simulink model "RMIC_ident_experiment"  (R2020a)
settings: Solver=ode4  StartTime=0.0  StopTime=30  FixedStep=1e-3  RelTol=1e-3
values from neighbouring files (symbols this model uses):
  lambdas = RMIC_get_fourier_lambdas(constPar.a_test, constPar.noj, constPar.nop, constPar.tend, constPar.omega, constPar.q_bound, constPar)    [RMIC_ident_experiment_start.m]
  q_dist_var = (pi*0.005/2)^2    (= 6.16850275068e-05)    [RMIC_ident_experiment_start.m]
  seed = 0    [RMIC_ident_experiment_start.m]
  T_smp = 1E-3    (= 0.001)    [RMIC_ident_experiment_start.m]
undefined symbols (not defined in the file or in its folder): constPar, f_c, f_nu, g, I1zz, I2zz, l1, lc1, lc2, m1, m2
settings Model: Creator=Tenghu  LastModifiedBy=fernando
settings SolverCC: ZeroCrossControl=EnableAll  AlgebraicLoopSolver=LineSearch
settings DataIOCC: SaveFormat=StructureWithTime
settings OptimizationCC: BlockReduction=off  BooleanDataType=off  LifeSpan=inf
settings DebuggingCC: SaveWithParameterizedLinksMsg=none  UnderspecifiedInitializationDetection=Classic  MergeDetectMultiDrivingBlocksExec=none  SignalResolutionControl=TryResolveAllWithWarning  AllowSymbolicDim=off  SFUnexpectedBacktrackingDiag=warning  SFNoUnconditionalDefaultTransitionDiag=warning  SFExecutionAtInitializationDiag=none  ArithmeticOperatorsInVariantConditions=warning
settings HardwareCC: ProdBitPerPointer=32  ProdBitPerSizeT=32  ProdBitPerPtrDiffT=32  ProdLargestAtomicFloat=None  ProdIntDivRoundTo=Undefined  ProdEndianess=Unspecified  ProdWordSize=32  ProdHWDeviceType=32-bit Generic  TargetBitPerLong=64  TargetBitPerPointer=64  TargetBitPerSizeT=64  TargetBitPerPtrDiffT=64  TargetLongLongMode=on  TargetIntDivRoundTo=Zero  TargetEndianess=LittleEndian  TargetWordSize=64  TargetHWDeviceType=MATLAB Host  ProdEqTarget=off
settings ModelReferenceCC: PropagateSignalLabelsOutOfModel=off
settings SFSimCC: SimUseLocalCustomCode=off  CustomCodeUndefinedFunction=UseInterfaceOnly
settings RTWCC: RTWUseLocalCustomCode=off
settings CodeAppCC: StateflowObjectComments=on
settings GRTTargetCC: TargetLangStandard=C89/C90 (ANSI)
settings ConfigComp: CovMetricSettings=dw  CovHtmlReporting=on  CovSaveCumulativeToWorkspaceVar=on  CovSaveSingleToWorkspaceVar=on  CovExternalEMLEnable=off  CovSFcnEnable=off

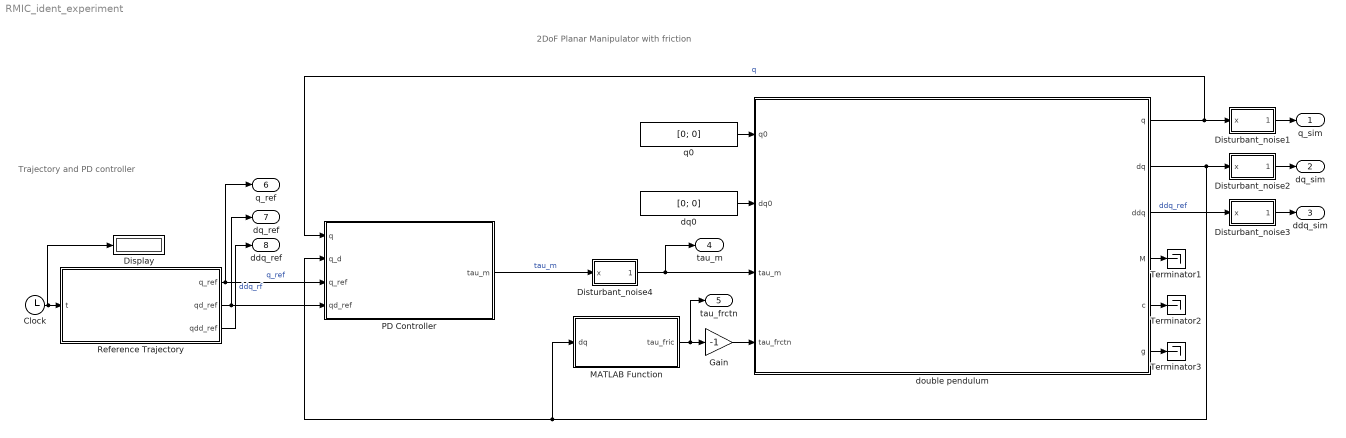
== system RMIC_ident_experiment ==
  note: Trajectory and PD controller
  note: 2DoF Planar Manipulator with friction
  Clock : Clock
  Display : Display
  Disturbant_noise1 : Subsystem  mask{q_dist_var=q_dist_var*100}
      mask prompts: q_dist_var "Varaiance of noise [rad^2]"
  Disturbant_noise2 : Subsystem  mask{q_dist_var=q_dist_var*100*2*pi}
      mask prompts: q_dist_var "Varaiance of noise [rad^2]"
  Disturbant_noise3 : Subsystem  mask{q_dist_var=q_dist_var*100*6*pi^2}
      mask prompts: q_dist_var "Varaiance of noise [rad^2]"
  Disturbant_noise4 : Subsystem  mask{q_dist_var=1.5^2}
      mask prompts: q_dist_var "Varaiance of noise [rad^2]"
  Gain : Gain  Gain=-1
  MATLAB Function : MATLAB Function  TreatAsAtomicUnit=on
  PD Controller : Subsystem
      mask Display:
      | image(imread('./controller.png'))
      | port_label('input', 1, 'q','interpreter','tex')
      | port_label('input', 2, 'dq','interpreter','tex')
      | port_label('input', 3, 'q_{ref}','interpreter','tex')
      | port_label('input', 4, 'dq_{ref}','interpreter','tex')
      | port_label('output', 1, '\tau_m','interpreter','tex')
  Reference Trajectory : Subsystem
      mask Display:
      | image(imread('./trajectory.png'))
      | port_label('input', 1, 't','interpreter','tex')
      | port_label('output', 1, 'q_{ref}','interpreter','tex')
      | port_label('output', 2, 'dq{ref}','interpreter','tex')
      | port_label('output', 3, 'ddq{ref}','interpreter','tex')
  Terminator1 : Terminator
  Terminator2 : Terminator
  Terminator3 : Terminator
  double pendulum : Subsystem
      mask Display:
      | image(imread('./double_pendulum.png'))
      | port_label('input', 1, 'q_0','interpreter','tex')
      | port_label('input', 2, 'dq_0','interpreter','tex')
      | port_label('input', 3, 'tau_{m}','interpreter','tex')
      | port_label('input', 4, 'tau_{frctn}','interpreter','tex')
      | 
      | port_label('output', 1, 'q','interpreter','tex')
      | port_label('output', 2, 'dq','interpreter','tex')
      | port_label('output', 3, 'ddq','interpreter','tex')
      | port_label('output', 4, 'M(q)','interpreter','tex')
      | port_label('output', 5, 'c(q,dq)','interpreter','tex')
      | port_label('output', 6, 'g(q)')
  dq0 : Constant  Value=[0; 0]
  q0 : Constant  Value=[0; 0]
  q_sim : Outport  VectorParamsAs1DForOutWhenUnconnected=off
  dq_sim : Outport  Port=2  VectorParamsAs1DForOutWhenUnconnected=off
  ddq_sim : Outport  Port=3  VectorParamsAs1DForOutWhenUnconnected=off
  tau_m : Outport  Port=4  VectorParamsAs1DForOutWhenUnconnected=off
  tau_frctn : Outport  Port=5  VectorParamsAs1DForOutWhenUnconnected=off
  q_ref : Outport  Port=6  VectorParamsAs1DForOutWhenUnconnected=off
  dq_ref : Outport  Port=7  VectorParamsAs1DForOutWhenUnconnected=off
  ddq_ref : Outport  Port=8  VectorParamsAs1DForOutWhenUnconnected=off
  wires:
  double pendulum/4(M) -> Terminator1/1
  double pendulum/5(c) -> Terminator2/1
  double pendulum/6(g) -> Terminator3/1
  dq0/1 -> double pendulum/2(dq0)
  q0/1 -> double pendulum/1(q0)
  Clock/1 -> Display/1, Reference Trajectory/1(t)
  MATLAB Function/1(tau_fric) -> tau_frctn/1, Gain/1
  double pendulum/3(ddq) -> Disturbant_noise3/1(x)  "ddq_ref"
  double pendulum/2(dq) -> Disturbant_noise2/1(x), MATLAB Function/1(dq), PD Controller/2(q_d)
  Gain/1 -> double pendulum/4(tau_frctn)
  PD Controller/1(tau_m) -> Disturbant_noise4/1(x)  "tau_m"
  double pendulum/1(q) -> Disturbant_noise1/1(x), PD Controller/1(q)  "q"
  Disturbant_noise2/1(x_dist) -> dq_sim/1
  Disturbant_noise1/1(x_dist) -> q_sim/1
  Disturbant_noise3/1(x_dist) -> ddq_sim/1
  Disturbant_noise4/1(x_dist) -> tau_m/1, double pendulum/3(tau_m)
  Reference Trajectory/3(qdd_ref) -> ddq_ref/1  "ddq_rf"
  Reference Trajectory/1(q_ref) -> q_ref/1, PD Controller/3(q_ref)  "q_ref"
  Reference Trajectory/2(qd_ref) -> dq_ref/1, PD Controller/4(qd_ref)

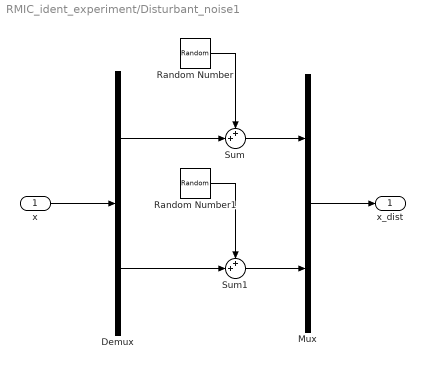
== system RMIC_ident_experiment/Disturbant_noise1 ==
  x : Inport
  Demux : Demux  Outputs=2
  Mux : Mux  Inputs=2
  Random Number : RandomNumber  Variance=q_dist_var  Seed=seed  SampleTime=T_smp
  Random Number1 : RandomNumber  Variance=q_dist_var  Seed=seed  SampleTime=T_smp
  Sum : Sum  Inputs=++|
  Sum1 : Sum  Inputs=++|
  x_dist : Outport  VectorParamsAs1DForOutWhenUnconnected=off
  wires:
  Sum/1 -> Mux/1
  Sum1/1 -> Mux/2
  Mux/1 -> x_dist/1
  x/1 -> Demux/1
  Random Number1/1 -> Sum1/1
  Random Number/1 -> Sum/1
  Demux/1 -> Sum/2
  Demux/2 -> Sum1/2

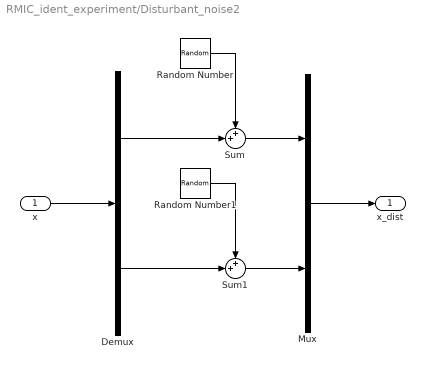
== system RMIC_ident_experiment/Disturbant_noise2 ==
  x : Inport
  Demux : Demux  Outputs=2
  Mux : Mux  Inputs=2
  Random Number : RandomNumber  Variance=q_dist_var  Seed=seed  SampleTime=T_smp
  Random Number1 : RandomNumber  Variance=q_dist_var  Seed=seed  SampleTime=T_smp
  Sum : Sum  Inputs=++|
  Sum1 : Sum  Inputs=++|
  x_dist : Outport  VectorParamsAs1DForOutWhenUnconnected=off
  wires:
  Sum/1 -> Mux/1
  Sum1/1 -> Mux/2
  Mux/1 -> x_dist/1
  x/1 -> Demux/1
  Random Number1/1 -> Sum1/1
  Random Number/1 -> Sum/1
  Demux/1 -> Sum/2
  Demux/2 -> Sum1/2

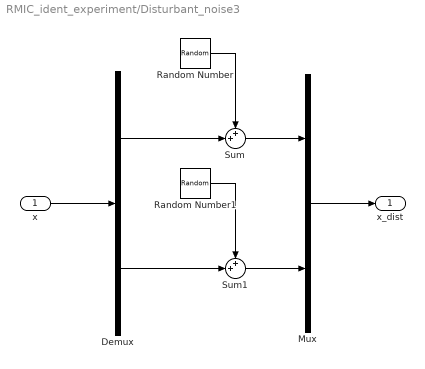
== system RMIC_ident_experiment/Disturbant_noise3 ==
  x : Inport
  Demux : Demux  Outputs=2
  Mux : Mux  Inputs=2
  Random Number : RandomNumber  Variance=q_dist_var  Seed=seed  SampleTime=T_smp
  Random Number1 : RandomNumber  Variance=q_dist_var  Seed=seed  SampleTime=T_smp
  Sum : Sum  Inputs=++|
  Sum1 : Sum  Inputs=++|
  x_dist : Outport  VectorParamsAs1DForOutWhenUnconnected=off
  wires:
  Sum/1 -> Mux/1
  Sum1/1 -> Mux/2
  Mux/1 -> x_dist/1
  x/1 -> Demux/1
  Random Number1/1 -> Sum1/1
  Random Number/1 -> Sum/1
  Demux/1 -> Sum/2
  Demux/2 -> Sum1/2

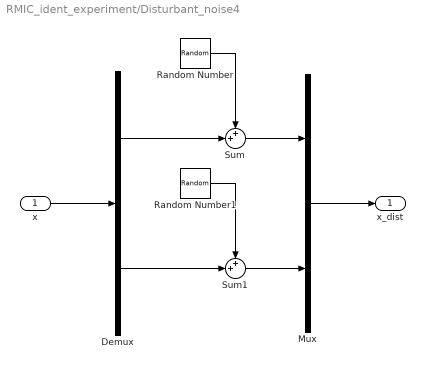
== system RMIC_ident_experiment/Disturbant_noise4 ==
  x : Inport
  Demux : Demux  Outputs=2
  Mux : Mux  Inputs=2
  Random Number : RandomNumber  Variance=q_dist_var  Seed=seed  SampleTime=T_smp
  Random Number1 : RandomNumber  Variance=q_dist_var  Seed=seed  SampleTime=T_smp
  Sum : Sum  Inputs=++|
  Sum1 : Sum  Inputs=++|
  x_dist : Outport  VectorParamsAs1DForOutWhenUnconnected=off
  wires:
  Demux/1 -> Sum/2
  Sum/1 -> Mux/1
  Demux/2 -> Sum1/2
  Sum1/1 -> Mux/2
  Random Number1/1 -> Sum1/1
  x/1 -> Demux/1
  Mux/1 -> x_dist/1
  Random Number/1 -> Sum/1

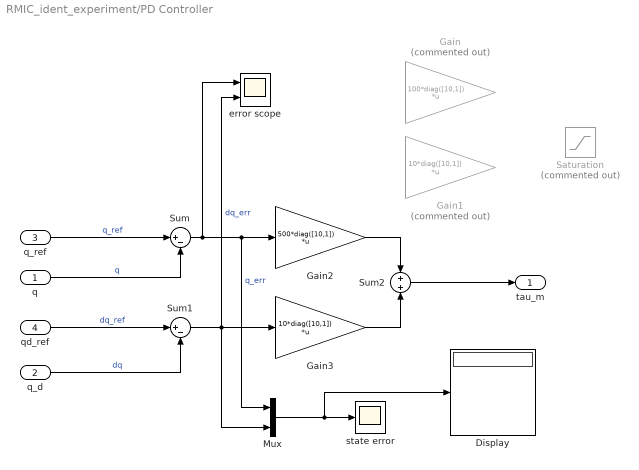
== system RMIC_ident_experiment/PD Controller ==
  q : Inport
  q_d : Inport  Port=2
  q_ref : Inport  Port=3
  qd_ref : Inport  Port=4
  Display : Display
  Gain : Gain  Commented=on  Gain=100*diag([10,1])  Multiplication=Matrix(K*u)
  Gain1 : Gain  Commented=on  Gain=10*diag([10,1])  Multiplication=Matrix(K*u)
  Gain2 : Gain  Gain=500*diag([10,1])  Multiplication=Matrix(K*u)
  Gain3 : Gain  Gain=10*diag([10,1])  Multiplication=Matrix(K*u)
  Mux : Mux  Inputs=2
  Saturation : Saturate  Commented=on  UpperLimit=constPar.maxTorque  LowerLimit=constPar.minTorque
  Sum : Sum  Inputs=|+-
  Sum1 : Sum  Inputs=|+-
  Sum2 : Sum
  error scope : Scope  NumInputPorts=2
  state error : Scope
  tau_m : Outport  VectorParamsAs1DForOutWhenUnconnected=off
  wires:
  q_ref/1 -> Sum/1  "q_ref"
  Sum/1 -> error scope/1, Gain2/1, Mux/1  "q_err"
  Sum1/1 -> Gain3/1, Mux/2, error scope/2  "dq_err"
  q/1 -> Sum/2  "q"
  q_d/1 -> Sum1/2  "dq"
  Mux/1 -> Display/1, state error/1
  Gain2/1 -> Sum2/1
  Gain3/1 -> Sum2/2
  Sum2/1 -> tau_m/1
  qd_ref/1 -> Sum1/1  "dq_ref"

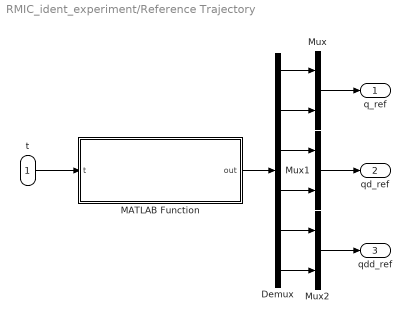
== system RMIC_ident_experiment/Reference Trajectory ==
  t : Inport
  Demux : Demux  Outputs=6
  MATLAB Function : MATLAB Function  TreatAsAtomicUnit=on
  Mux : Mux  Inputs=2
  Mux1 : Mux  Inputs=2
  Mux2 : Mux  Inputs=2
  q_ref : Outport  VectorParamsAs1DForOutWhenUnconnected=off
  qd_ref : Outport  Port=2  VectorParamsAs1DForOutWhenUnconnected=off
  qdd_ref : Outport  Port=3  VectorParamsAs1DForOutWhenUnconnected=off
  wires:
  t/1 -> MATLAB Function/1(t)
  Demux/1 -> Mux/1
  Demux/2 -> Mux/2
  Demux/3 -> Mux1/1
  Demux/4 -> Mux1/2
  Demux/5 -> Mux2/1
  Demux/6 -> Mux2/2
  MATLAB Function/1(out) -> Demux/1
  Mux/1 -> q_ref/1
  Mux1/1 -> qd_ref/1
  Mux2/1 -> qdd_ref/1

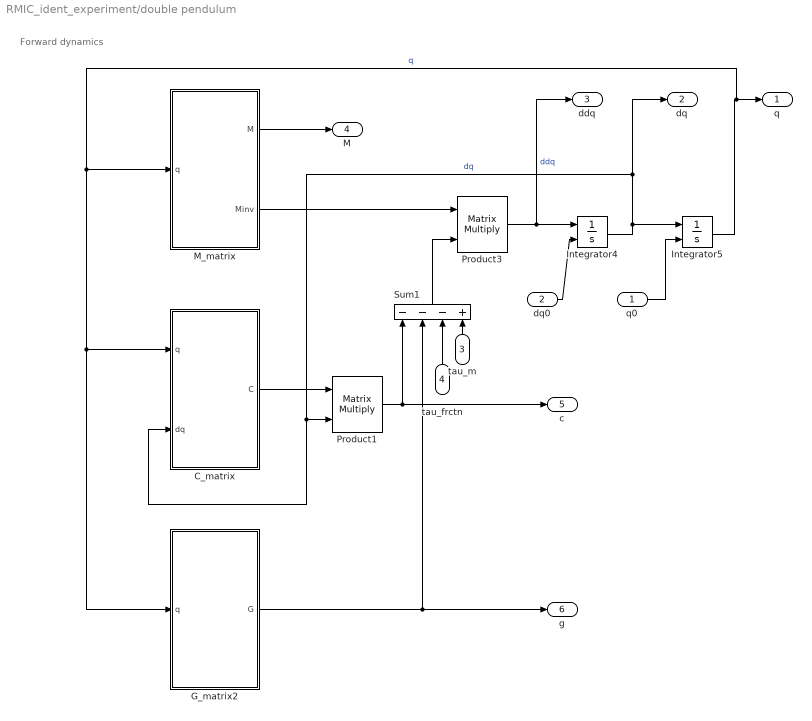
== system RMIC_ident_experiment/double pendulum ==
  note: Forward dynamics
  q0 : Inport
  dq0 : Inport  Port=2
  tau_m : Inport  Port=3
  tau_frctn : Inport  Port=4
  C_matrix : MATLAB Function  TreatAsAtomicUnit=on
  G_matrix2 : MATLAB Function  TreatAsAtomicUnit=on
  Integrator4 : Integrator  InitialConditionSource=external  InitialCondition=[0,0]
  Integrator5 : Integrator  InitialConditionSource=external
  M_matrix : MATLAB Function  TreatAsAtomicUnit=on
  Product1 : Product  Multiplication=Matrix(*)
  Product3 : Product  Multiplication=Matrix(*)
  Sum1 : Sum  Inputs=---+
  q : Outport  VectorParamsAs1DForOutWhenUnconnected=off
  dq : Outport  Port=2  VectorParamsAs1DForOutWhenUnconnected=off
  ddq : Outport  Port=3  VectorParamsAs1DForOutWhenUnconnected=off
  M : Outport  Port=4  VectorParamsAs1DForOutWhenUnconnected=off
  c : Outport  Port=5  VectorParamsAs1DForOutWhenUnconnected=off
  g : Outport  Port=6  VectorParamsAs1DForOutWhenUnconnected=off
  wires:
  M_matrix/2(Minv) -> Product3/1
  Product3/1 -> ddq/1, Integrator4/1  "ddq"
  C_matrix/1(C) -> Product1/1
  Product1/1 -> Sum1/1, c/1
  Integrator5/1 -> C_matrix/1(q), G_matrix2/1(q), M_matrix/1(q), q/1  "q"
  Integrator4/1 -> Integrator5/1, dq/1, Product1/2, C_matrix/2(dq)  "dq"
  G_matrix2/1(G) -> Sum1/2, g/1
  q0/1 -> Integrator5/2
  M_matrix/1(M) -> M/1
  tau_m/1 -> Sum1/4
  Sum1/1 -> Product3/2
  tau_frctn/1 -> Sum1/3
  dq0/1 -> Integrator4/2

== matlab function RMIC_ident_experiment/Reference Trajectory/MATLAB Function ==
  data: t input; out output; constPar parameter; lambdas parameter
function out = fcn_twoLink_refOptTrajectory(t, constPar, lambdas)
    
    Q = zeros(6,1);
    if(constPar.test_trajectory)
        param           = constPar.a_test;
    else
        param           = constPar.a_opt;   
    end
    noj=2;
    omega           = constPar.omega;
    constPar.n_cos = numel(param)/noj;
    n_cos  = constPar.n_cos;
   
    a_im = zeros(2,5); % Parameters from eq. (35)
    for i = 1:noj
        a_im(i,:) = (param(1+(i-1)*constPar.n_cos:constPar.n_cos+(i-1)*constPar.n_cos))'; 
    end

    
    tf = 2*pi/omega;            
    if t > tf
        t = t - tf*fix(t/tf);
    end

    delta    = zeros(1,noj);
    D_delta  = zeros(1,noj);
    DD_delta = zeros(1,noj);  
    
    lambda_poly   = zeros(1,noj);
    dlambda_poly  = zeros(1,noj);
    ddlambda_poly = zeros(1,noj);   
    
    for j = 1:noj
        delta_    = 0;
        D_delta_  = 0;
        DD_delta_ = 0;
        for mf = 1:n_cos
          delta_    =    delta_ + a_im(j,mf)*cos((mf*pi/tf)*t);
          D_delta_  =  D_delta_ - a_im(j,mf)*sin((mf*pi/tf)*t)*(mf*pi/tf);
          DD_delta_ = DD_delta_ - a_im(j,mf)*cos((mf*pi/tf)*t)*(mf*pi/tf)^2;
        end
        delta(1,j)         = delta_;
        D_delta(1,j)       = D_delta_;
        DD_delta(1,j)      = DD_delta_;
        lambda_poly(1,j)   = polyval(flip(lambdas(:,j)'),t)';
        dlambda_poly(1,j)  = polyval(polyder(flip(lambdas(:,j)')),t)';
        ddlambda_poly(1,j) = polyval(polyder(polyder(flip(lambdas(:,j)'))),t)';  
    end
    q   = delta    + lambda_poly;
    qD  = D_delta  + dlambda_poly;
    qDD = DD_delta + ddlambda_poly;
    Q = [q';qD';qDD'];
   out = Q;%zeros(6,1);
end

== matlab function RMIC_ident_experiment/MATLAB Function ==
  data: dq input; tau_fric output; f_nu parameter; f_c parameter; constPar parameter
function tau_fric = fcn_friction_twoLink(dq, f_nu, f_c, constPar)
    fvis = f_nu*eye(2)*dq;

    if constPar.useCoulomb  % A continuous friction model to ease the simulation
        tau_fric = fvis + f_c*eye(2)*tanh(constPar.tanh_coef*dq);
    else
        tau_fric = fvis;
    end
end

== matlab function RMIC_ident_experiment/double pendulum/C_matrix ==
  data: q input; C output; dq input; l1 parameter; lc2 parameter; m2 parameter
function C = C_matrix(q,dq, l1, lc2, m2)
%#codegen

%    This function was generated by the Symbolic Math Toolbox version 8.3.
%    05-Nov-2019 15:18:30

dq1  = dq(1);
dq2  = dq(2);
q1   = q(1);
q2   = q(2);

t2 = sin(q2);
C = reshape([-dq2.*l1.*lc2.*m2.*t2,dq1.*l1.*lc2.*m2.*t2,-l1.*lc2.*m2.*t2.*(dq1+dq2),0.0],[2,2]);

== matlab function RMIC_ident_experiment/double pendulum/G_matrix2 ==
  data: G output; q input; g parameter; l1 parameter; lc1 parameter; lc2 parameter; m1 parameter; m2 parameter
function G = G_matrix(q, g, l1, lc1, lc2, m1, m2)
%#codegen

%    This function was generated by the Symbolic Math Toolbox version 8.3.
%    05-Nov-2019 15:18:30

q1   = q(1);
q2   = q(2);

t2 = cos(q1);
t3 = q1+q2;
t4 = cos(t3);
G = [g.*m2.*(l1.*t2+lc2.*t4)+g.*lc1.*m1.*t2;g.*lc2.*m2.*t4];

== matlab function RMIC_ident_experiment/double pendulum/M_matrix ==
  data: M output; q input; I1zz parameter; I2zz parameter; l1 parameter; lc1 parameter; lc2 parameter; m1 parameter; m2 parameter; Minv output
function [M, Minv] = M_matrix(q, I1zz, I2zz, l1, lc1, lc2, m1, m2)
%#codegen

%    This function was generated by the Symbolic Math Toolbox version 8.3.
%    05-Nov-2019 15:18:29

q1   = q(1);
q2   = q(2);

t2 = cos(q2);
t3 = lc2.^2;
t4 = m2.*t3;
t5 = l1.*lc2.*m2.*t2;
t6 = I2zz+t4+t5;
M = reshape([I1zz+t5+t6+l1.^2.*m2+lc1.^2.*m1,t6,t6,I2zz+t4],[2,2]);
Minv = pinv(M);
